simulink library "CTC_lib"  (Simulink 7.4)
settings: Solver=ode45  StartTime=0.0  StopTime=10.0  RelTol=1e-3
values from neighbouring files (symbols this model uses):
  CTCc_cnt_PrecGradVoltDeb = mpt.Parameter    [CTC_CAL.m]
  CTCc_i_HVCnctCur_max = mpt.Parameter    [CTC_CAL.m]
  CTCc_i_HVDcnctCur_max = mpt.Parameter    [CTC_CAL.m]
  CTCc_i_HVDcncWaitCur_max = mpt.Parameter    [CTC_CAL.m]
  CTCc_i_PrecCur_max = mpt.Parameter    [CTC_CAL.m]
  CTCc_pct_HVCnctTarVolt = mpt.Parameter    [CTC_CAL.m]
  CTCc_pct_HVDcnctTarVolt = mpt.Parameter    [CTC_CAL.m]
  CTCc_pct_NegCtrDiagCld = mpt.Parameter    [CTC_CAL.m]
  CTCc_pct_NegCtrDiagOpen = mpt.Parameter    [CTC_CAL.m]
  CTCc_pct_PosCtrDiagCld = mpt.Parameter    [CTC_CAL.m]
  CTCc_pct_PosCtrDiagOpen = mpt.Parameter    [CTC_CAL.m]
  CTCc_pct_PrecTarVolt = mpt.Parameter    [CTC_CAL.m]
  CTCc_pct_PrecVoltAllow = mpt.Parameter    [CTC_CAL.m]
  CTCc_tm_CtrClsCheckDly = mpt.Parameter    [CTC_CAL.m]
  CTCc_tm_CtrClsCheckDly_max = mpt.Parameter    [CTC_CAL.m]
  CTCc_tm_CtrOpenCheck_max = mpt.Parameter    [CTC_CAL.m]
  CTCc_tm_CtrOpenCheckDly = mpt.Parameter    [CTC_CAL.m]
  CTCc_tm_HVCnctTm_max = mpt.Parameter    [CTC_CAL.m]
  CTCc_tm_HVDcnctTm_max = mpt.Parameter    [CTC_CAL.m]
  CTCc_tm_HVDcnctWaitTm = mpt.Parameter    [CTC_CAL.m]
  CTCc_tm_HVDcnctWaitTm_max = mpt.Parameter    [CTC_CAL.m]
  CTCc_tm_HVEmcyDcnctTm_max = mpt.Parameter    [CTC_CAL.m]
  CTCc_tm_PrecTm_max = mpt.Parameter    [CTC_CAL.m]
  CTCc_tm_PrecVoltAlow = mpt.Parameter    [CTC_CAL.m]
  CTCc_tm_Tick_s = mpt.Parameter    [CTC_CAL.m]
  CTCc_v_PrecGradVolt = mpt.Parameter    [CTC_CAL.m]
  CTCc_v_PrecTarVoltDif = mpt.Parameter    [CTC_CAL.m]
libraries: Defined_Functionality x4
(part 1 of 2)
Description:
  | $Author:Zhao XiangRi$
  | $Date:2015/03/26$
  | $Revision:1.0$
settings Model: Creator=lixuying  LastModifiedBy=sunsijun

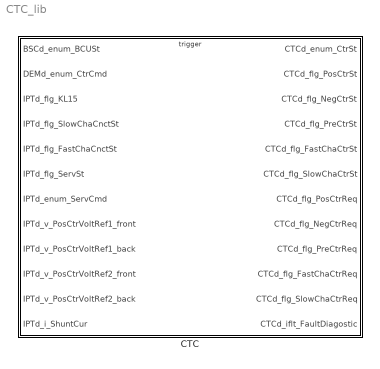
== system CTC_lib ==
  CTC : Subsystem  TreatAsAtomicUnit=on
      settings: RTWFcnNameOpts=Use subsystem name  RTWFileNameOpts=Use function name

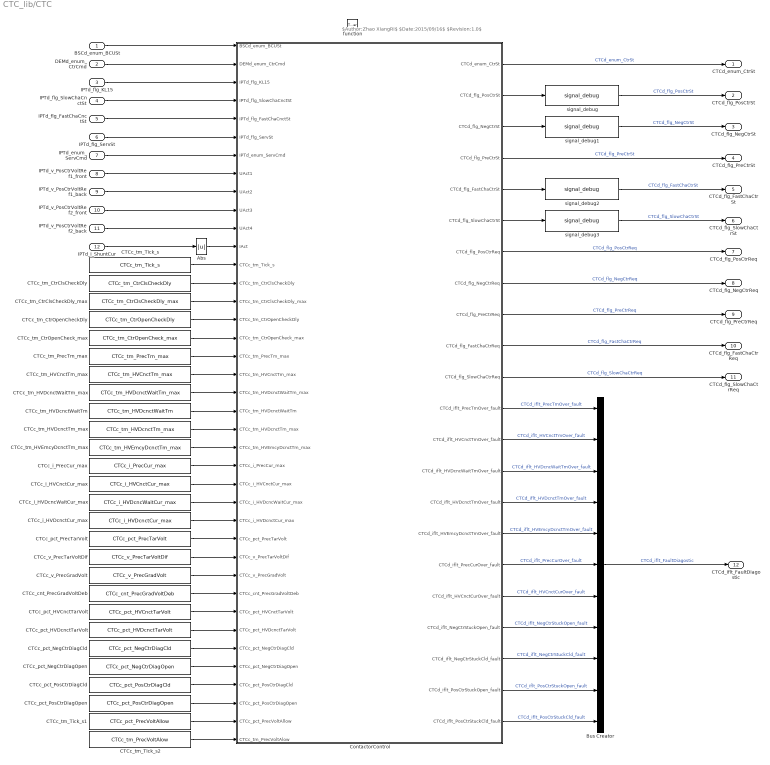
== system CTC_lib/CTC ==
  note: $Author:Zhao XiangRi$
      | $Date:2015/09/16$
      | $Revision:1.0$
  BSCd_enum_BCUSt : Inport
  DEMd_enum_CtrCmd : Inport  Port=2
  IPTd_flg_KL15 : Inport  Port=3  OutDataType=fixdt(1, 16)  OutScaling=2^0
  IPTd_flg_SlowChaCnctSt : Inport  Port=4  OutDataType=fixdt(1, 16)  OutScaling=2^0
  IPTd_flg_FastChaCnctSt : Inport  Port=5  OutDataType=fixdt(1, 16)  OutScaling=2^0
  IPTd_flg_ServSt : Inport  Port=6  OutDataType=fixdt(1, 16)  OutScaling=2^0
  IPTd_enum_ServCmd : Inport  Port=7
  IPTd_v_PosCtrVoltRef1_front : Inport  Port=8
  IPTd_v_PosCtrVoltRef1_back : Inport  Port=9
  IPTd_v_PosCtrVoltRef2_front : Inport  Port=10
  IPTd_v_PosCtrVoltRef2_back : Inport  Port=11
  IPTd_i_ShuntCur : Inport  Port=12
  function : TriggerPort  TriggerType=function-call
  Abs : Abs
  Bus Creator : BusCreator  Inputs=11
  CTCc_cnt_PrecGradVoltDeb : Constant  Value=CTCc_cnt_PrecGradVoltDeb
  CTCc_i_HVCnctCur_max : Constant  Value=CTCc_i_HVCnctCur_max
  CTCc_i_HVDcncWaitCur_max : Constant  Value=CTCc_i_HVDcncWaitCur_max
  CTCc_i_HVDcnctCur_max : Constant  Value=CTCc_i_HVDcnctCur_max
  CTCc_i_PrecCur_max : Constant  Value=CTCc_i_PrecCur_max
  CTCc_pct_HVCnctTarVolt : Constant  Value=CTCc_pct_HVCnctTarVolt
  CTCc_pct_HVDcnctTarVolt : Constant  Value=CTCc_pct_HVDcnctTarVolt
  CTCc_pct_NegCtrDiagCld : Constant  Value=CTCc_pct_NegCtrDiagCld
  CTCc_pct_NegCtrDiagOpen : Constant  Value=CTCc_pct_NegCtrDiagOpen
  CTCc_pct_PosCtrDiagCld : Constant  Value=CTCc_pct_PosCtrDiagCld
  CTCc_pct_PosCtrDiagOpen : Constant  Value=CTCc_pct_PosCtrDiagOpen
  CTCc_pct_PrecTarVolt : Constant  Value=CTCc_pct_PrecTarVolt
  CTCc_tm_CtrClsCheckDly : Constant  Value=CTCc_tm_CtrClsCheckDly
  CTCc_tm_CtrClsCheckDly_max : Constant  Value=CTCc_tm_CtrClsCheckDly_max
  CTCc_tm_CtrOpenCheckDly : Constant  Value=CTCc_tm_CtrOpenCheckDly
  CTCc_tm_CtrOpenCheck_max : Constant  Value=CTCc_tm_CtrOpenCheck_max
  CTCc_tm_HVCnctTm_max : Constant  Value=CTCc_tm_HVCnctTm_max
  CTCc_tm_HVDcnctTm_max : Constant  Value=CTCc_tm_HVDcnctTm_max
  CTCc_tm_HVDcnctWaitTm : Constant  Value=CTCc_tm_HVDcnctWaitTm
  CTCc_tm_HVDcnctWaitTm_max : Constant  Value=CTCc_tm_HVDcnctWaitTm_max
  CTCc_tm_HVEmcyDcnctTm_max : Constant  Value=CTCc_tm_HVEmcyDcnctTm_max
  CTCc_tm_PrecTm_max : Constant  Value=CTCc_tm_PrecTm_max
  CTCc_tm_Tick_s : Constant  Value=CTCc_tm_Tick_s  OutDataTypeMode=single  OutDataTypeStr=single
  CTCc_tm_Tick_s1 : Constant  Value=CTCc_pct_PrecVoltAllow  OutDataTypeMode=single  OutDataTypeStr=single
  CTCc_tm_Tick_s2 : Constant  Value=CTCc_tm_PrecVoltAlow  OutDataTypeMode=single  OutDataTypeStr=single
  CTCc_v_PrecGradVolt : Constant  Value=CTCc_v_PrecGradVolt
  CTCc_v_PrecTarVoltDif : Constant  Value=CTCc_v_PrecTarVoltDif
  ContactorControl : Stateflow chart  Description=|  TreatAsAtomicUnit=on
      | $Author:Zhao XiangRi$
      | $Date:2015/03/26$    
      | $Revision:1.0$
  signal_debug : Defined_Functionality/signal_debug  SystemSampleTime=-1  debug_switch=CTCc_dbgsw_PosCtrSt  debug_value=CTCc_dbgval_PosCtrSt
      settings: AttributesFormatString=[SWITCH=%<debug_switch>]\n[VALUE=%<debug_value>]
  signal_debug1 : Defined_Functionality/signal_debug  SystemSampleTime=-1  debug_switch=CTCc_dbgsw_NegCtrSt  debug_value=CTCc_dbgval_NegCtrSt
      settings: AttributesFormatString=[SWITCH=%<debug_switch>]\n[VALUE=%<debug_value>]
  signal_debug2 : Defined_Functionality/signal_debug  SystemSampleTime=-1  debug_switch=CTCc_dbgsw_FastChaCtrSt  debug_value=CTCc_dbgval_FastChaCtrSt
      settings: AttributesFormatString=[SWITCH=%<debug_switch>]\n[VALUE=%<debug_value>]
  signal_debug3 : Defined_Functionality/signal_debug  SystemSampleTime=-1  debug_switch=CTCc_dbgsw_SlowChaCtrSt  debug_value=CTCc_dbgval_SlowChaCtrSt
      settings: AttributesFormatString=[SWITCH=%<debug_switch>]\n[VALUE=%<debug_value>]
  CTCd_enum_CtrSt : Outport
  CTCd_flg_PosCtrSt : Outport  Port=2
  CTCd_flg_NegCtrSt : Outport  Port=3
  CTCd_flg_PreCtrSt : Outport  Port=4
  CTCd_flg_FastChaCtrSt : Outport  Port=5
  CTCd_flg_SlowChaCtrSt : Outport  Port=6
  CTCd_flg_PosCtrReq : Outport  Port=7
  CTCd_flg_NegCtrReq : Outport  Port=8
  CTCd_flg_PreCtrReq : Outport  Port=9
  CTCd_flg_FastChaCtrReq : Outport  Port=10
  CTCd_flg_SlowChaCtrReq : Outport  Port=11
  CTCd_iflt_FaultDiagostic : Outport  Port=12
  wires:
  ContactorControl/22(CTCd_iflt_PosCtrStuckCld_fault) -> Bus Creator/11  "CTCd_iflt_PosCtrStuckCld_fault"
  ContactorControl/21(CTCd_iflt_PosCtrStuckOpen_fault) -> Bus Creator/10  "CTCd_iflt_PosCtrStuckOpen_fault"
  ContactorControl/20(CTCd_iflt_NegCtrStuckCld_fault) -> Bus Creator/9  "CTCd_iflt_NegCtrStuckCld_fault"
  ContactorControl/19(CTCd_iflt_NegCtrStuckOpen_fault) -> Bus Creator/8  "CTCd_iflt_NegCtrStuckOpen_fault"
  ContactorControl/18(CTCd_iflt_HVCnctCurOver_fault) -> Bus Creator/7  "CTCd_iflt_HVCnctCurOver_fault"
  ContactorControl/17(CTCd_iflt_PrecCurOver_fault) -> Bus Creator/6  "CTCd_iflt_PrecCurOver_fault"
  ContactorControl/16(CTCd_iflt_HVEmcyDcnctTmOver_fault) -> Bus Creator/5  "CTCd_iflt_HVEmcyDcnctTmOver_fault"
  ContactorControl/15(CTCd_iflt_HVDcnctTmOver_fault) -> Bus Creator/4  "CTCd_iflt_HVDcnctTmOver_fault"
  ContactorControl/14(CTCd_iflt_HVDcncWaitTmOver_fault) -> Bus Creator/3  "CTCd_iflt_HVDcncWaitTmOver_fault"
  ContactorControl/13(CTCd_iflt_HVCnctTmOver_fault) -> Bus Creator/2  "CTCd_iflt_HVCnctTmOver_fault"
  ContactorControl/12(CTCd_iflt_PrecTmOver_fault) -> Bus Creator/1  "CTCd_iflt_PrecTmOver_fault"
  Bus Creator/1 -> CTCd_iflt_FaultDiagostic/1  "CTCd_iflt_FaultDiagostic"
  DEMd_enum_CtrCmd/1 -> ContactorControl/2(DEMd_enum_CtrCmd)
  ContactorControl/11(CTCd_flg_SlowChaCtrReq) -> CTCd_flg_SlowChaCtrReq/1  "CTCd_flg_SlowChaCtrReq"
  ContactorControl/6(CTCd_flg_SlowChaCtrSt) -> signal_debug3/1
  ContactorControl/5(CTCd_flg_FastChaCtrSt) -> signal_debug2/1
  ContactorControl/7(CTCd_flg_PosCtrReq) -> CTCd_flg_PosCtrReq/1  "CTCd_flg_PosCtrReq"
  IPTd_v_PosCtrVoltRef2_back/1 -> ContactorControl/11(UAct4)
  CTCc_tm_Tick_s/1 -> ContactorControl/13(CTCc_tm_Tick_s)
  CTCc_pct_PosCtrDiagCld/1 -> ContactorControl/36(CTCc_pct_PosCtrDiagCld)
  CTCc_pct_PosCtrDiagOpen/1 -> ContactorControl/37(CTCc_pct_PosCtrDiagOpen)
  CTCc_pct_NegCtrDiagCld/1 -> ContactorControl/34(CTCc_pct_NegCtrDiagCld)
  CTCc_pct_NegCtrDiagOpen/1 -> ContactorControl/35(CTCc_pct_NegCtrDiagOpen)
  CTCc_pct_HVCnctTarVolt/1 -> ContactorControl/32(CTCc_pct_HVCnctTarVolt)
  CTCc_v_PrecTarVoltDif/1 -> ContactorControl/29(CTCc_v_PrecTarVoltDif)
  CTCc_pct_HVDcnctTarVolt/1 -> ContactorControl/33(CTCc_pct_HVDcnctTarVolt)
  CTCc_pct_PrecTarVolt/1 -> ContactorControl/28(CTCc_pct_PrecTarVolt)
  CTCc_i_HVDcnctCur_max/1 -> ContactorControl/27(CTCc_i_HVDcnctCur_max)
  CTCc_v_PrecGradVolt/1 -> ContactorControl/30(CTCc_v_PrecGradVolt)
  CTCc_cnt_PrecGradVoltDeb/1 -> ContactorControl/31(CTCc_cnt_PrecGradVoltDeb)
  ContactorControl/9(CTCd_flg_PreCtrReq) -> CTCd_flg_PreCtrReq/1  "CTCd_flg_PreCtrReq"
  ContactorControl/8(CTCd_flg_NegCtrReq) -> CTCd_flg_NegCtrReq/1  "CTCd_flg_NegCtrReq"
  ContactorControl/4(CTCd_flg_PreCtrSt) -> CTCd_flg_PreCtrSt/1  "CTCd_flg_PreCtrSt"
  ContactorControl/2(CTCd_flg_PosCtrSt) -> signal_debug/1
  ContactorControl/1(CTCd_enum_CtrSt) -> CTCd_enum_CtrSt/1  "CTCd_enum_CtrSt"
  ContactorControl/10(CTCd_flg_FastChaCtrReq) -> CTCd_flg_FastChaCtrReq/1  "CTCd_flg_FastChaCtrReq"
  ContactorControl/3(CTCd_flg_NegCtrSt) -> signal_debug1/1
  IPTd_i_ShuntCur/1 -> Abs/1
  IPTd_v_PosCtrVoltRef1_front/1 -> ContactorControl/8(UAct1)
  IPTd_v_PosCtrVoltRef1_back/1 -> ContactorControl/9(UAct2)
  IPTd_v_PosCtrVoltRef2_front/1 -> ContactorControl/10(UAct3)
  IPTd_enum_ServCmd/1 -> ContactorControl/7(IPTd_enum_ServCmd)
  CTCc_tm_CtrClsCheckDly/1 -> ContactorControl/14(CTCc_tm_CtrClsCheckDly)
  CTCc_tm_CtrClsCheckDly_max/1 -> ContactorControl/15(CTCc_tm_CtrClsCheckDly_max)
  CTCc_tm_CtrOpenCheckDly/1 -> ContactorControl/16(CTCc_tm_CtrOpenCheckDly)
  CTCc_tm_CtrOpenCheck_max/1 -> ContactorControl/17(CTCc_tm_CtrOpenCheck_max)
  CTCc_tm_PrecTm_max/1 -> ContactorControl/18(CTCc_tm_PrecTm_max)
  CTCc_tm_HVCnctTm_max/1 -> ContactorControl/19(CTCc_tm_HVCnctTm_max)
  CTCc_tm_HVDcnctWaitTm_max/1 -> ContactorControl/20(CTCc_tm_HVDcnctWaitTm_max)
  CTCc_tm_HVDcnctTm_max/1 -> ContactorControl/22(CTCc_tm_HVDcnctTm_max)
  CTCc_tm_HVEmcyDcnctTm_max/1 -> ContactorControl/23(CTCc_tm_HVEmcyDcnctTm_max)
  CTCc_i_PrecCur_max/1 -> ContactorControl/24(CTCc_i_PrecCur_max)
  CTCc_i_HVCnctCur_max/1 -> ContactorControl/25(CTCc_i_HVCnctCur_max)
  CTCc_i_HVDcncWaitCur_max/1 -> ContactorControl/26(CTCc_i_HVDcncWaitCur_max)
  CTCc_tm_HVDcnctWaitTm/1 -> ContactorControl/21(CTCc_tm_HVDcnctWaitTm)
  Abs/1 -> ContactorControl/12(IAct)
  BSCd_enum_BCUSt/1 -> ContactorControl/1(BSCd_enum_BCUSt)
  CTCc_tm_Tick_s1/1 -> ContactorControl/38(CTCc_pct_PrecVoltAllow)
  CTCc_tm_Tick_s2/1 -> ContactorControl/39(CTCc_tm_PrecVoltAlow)
  IPTd_flg_KL15/1 -> ContactorControl/3(IPTd_flg_KL15)
  IPTd_flg_SlowChaCnctSt/1 -> ContactorControl/4(IPTd_flg_SlowChaCnctSt)
  IPTd_flg_FastChaCnctSt/1 -> ContactorControl/5(IPTd_flg_FastChaCnctSt)
  IPTd_flg_ServSt/1 -> ContactorControl/6(IPTd_flg_ServSt)
  signal_debug/1 -> CTCd_flg_PosCtrSt/1  "CTCd_flg_PosCtrSt"
  signal_debug1/1 -> CTCd_flg_NegCtrSt/1  "CTCd_flg_NegCtrSt"
  signal_debug2/1 -> CTCd_flg_FastChaCtrSt/1  "CTCd_flg_FastChaCtrSt"
  signal_debug3/1 -> CTCd_flg_SlowChaCtrSt/1  "CTCd_flg_SlowChaCtrSt"
